simulink library "INT_EngPrt_PrtLimMech"  (R2016b)
settings: Solver=VariableStepAuto  StartTime=0.0  StopTime=10.0  RelTol=1e-3
settings Model: Creator=xuxingpei  LastModifiedBy=xuxingpei

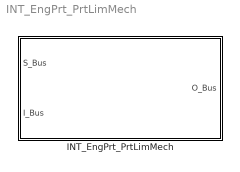
== system INT_EngPrt_PrtLimMech ==
  INT_EngPrt_PrtLimMech : Subsystem

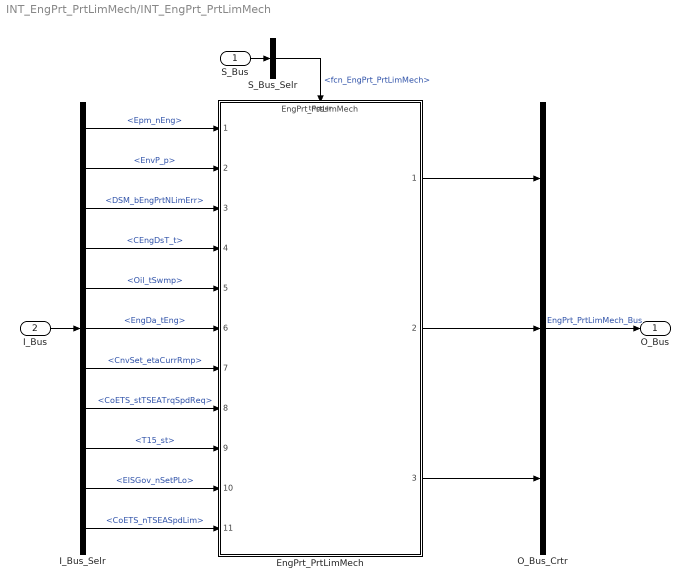
== system INT_EngPrt_PrtLimMech/INT_EngPrt_PrtLimMech ==
  S_Bus : Inport
  I_Bus : Inport  Port=2
  EngPrt_PrtLimMech : ModelReference  ModelNameDialog=EngPrt_PrtLimMech  SimulationMode=Normal  ModelReferenceVersion=1.43  TriggerPortName=function  TriggerPortTriggerType=function-call  TriggerPortStatesWhenEnabling=held
  I_Bus_Selr : BusSelector  OutputSignals=Epm_nEng,EnvP_p,DSM_bEngPrtNLimErr,CEngDsT_t,Oil_tSwmp,EngDa_tEng,CnvSet_etaCurrRmp,CoETS_stTSEATrqSpdReq,T15_st,EISGov_nSetPLo,CoETS_nTSEASpdLim
  O_Bus_Crtr : BusCreator  Inputs=3
  S_Bus_Selr : BusSelector  OutputSignals=fcn_EngPrt_PrtLimMech
  O_Bus : Outport
  wires:
  S_Bus_Selr/1 -> EngPrt_PrtLimMech/Trigger  "<fcn_EngPrt_PrtLimMech>"
  S_Bus/1 -> S_Bus_Selr/1
  I_Bus/1 -> I_Bus_Selr/1
  I_Bus_Selr/1 -> EngPrt_PrtLimMech/1  "<Epm_nEng>"
  I_Bus_Selr/2 -> EngPrt_PrtLimMech/2  "<EnvP_p>"
  I_Bus_Selr/3 -> EngPrt_PrtLimMech/3  "<DSM_bEngPrtNLimErr>"
  I_Bus_Selr/4 -> EngPrt_PrtLimMech/4  "<CEngDsT_t>"
  I_Bus_Selr/5 -> EngPrt_PrtLimMech/5  "<Oil_tSwmp>"
  I_Bus_Selr/6 -> EngPrt_PrtLimMech/6  "<EngDa_tEng>"
  I_Bus_Selr/7 -> EngPrt_PrtLimMech/7  "<CnvSet_etaCurrRmp>"
  I_Bus_Selr/8 -> EngPrt_PrtLimMech/8  "<CoETS_stTSEATrqSpdReq>"
  I_Bus_Selr/9 -> EngPrt_PrtLimMech/9  "<T15_st>"
  I_Bus_Selr/10 -> EngPrt_PrtLimMech/10  "<EISGov_nSetPLo>"
  I_Bus_Selr/11 -> EngPrt_PrtLimMech/11  "<CoETS_nTSEASpdLim>"
  O_Bus_Crtr/1 -> O_Bus/1  "EngPrt_PrtLimMech_Bus"
  EngPrt_PrtLimMech/1 -> O_Bus_Crtr/1
  EngPrt_PrtLimMech/2 -> O_Bus_Crtr/2
  EngPrt_PrtLimMech/3 -> O_Bus_Crtr/3
